simulink model "mloc_diag_vehicle"  (R2018b)
settings: configuration reference "Active" (kept outside this file)
undefined symbols (not defined in the file): P_MLOC_ActivateVehicleUnstableDetection_b, P_MLOC_BetaMax_rad, P_MLOC_SafeStandstill_FMax_N, P_MLOC_SafeStandstill_vabsMax_mps
libraries: simulink x3
settings Model: DataDictionary=mloc_diag_vehicle.sldd  Creator=wischnewski  LastModifiedBy=ge34qer

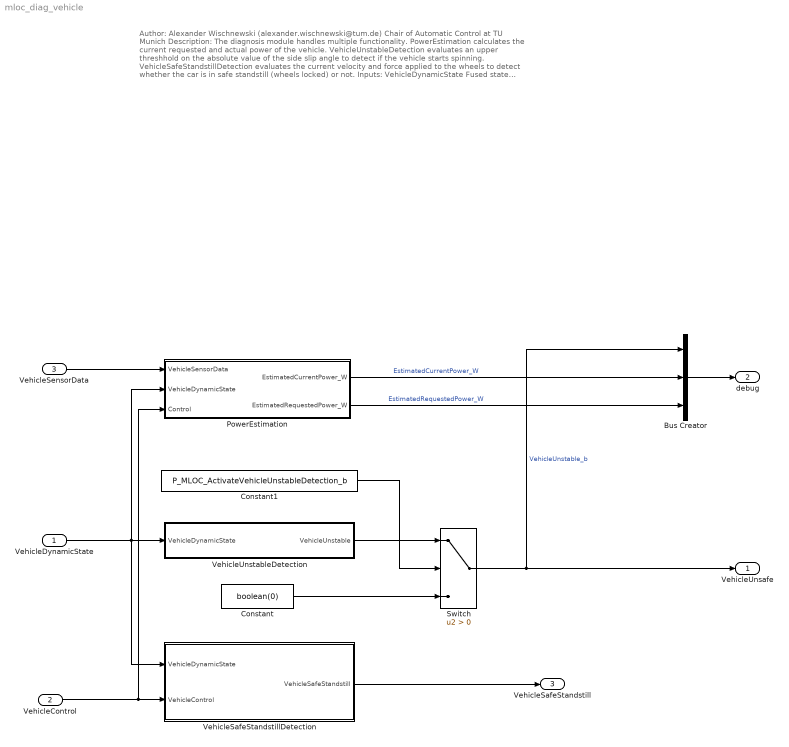
== system mloc_diag_vehicle ==
  note: Author: Alexander Wischnewski (alexander.wischnewski@tum.de)
      | Chair of Automatic Control at TU Munich
      |
      | Description: The diagnosis module handles multiple functionality.
      |
      | PowerEstimation calculates the current requested and actual power of the
      | vehicle.
      |
      | VehicleUnstableDetection evaluates an upper threshhold on the absolute value
      | of the side slip angle to detect if the vehicle starts spinning.
      |
      | VehicleSafeStandstillDetection evaluates the current velocity and force applied to the
      | wheels to detect whether the car is in safe standstill (wheels locked) or not.
      |
      | Inputs:
      | VehicleDynamicState Fused state vector of the vehicle (including position, velocity, acceleration, etc.)
      | VehicleControl Low level vehicle controller output
      | VehicleSensorData Raw sensor data of all vehicle sensors
      |
      | Outputs:
      | debug All debug values
      | VehicleUnsafe Safety critical diagnosis triggered
      | VehicleSafeStandstill Safe standstill detected
  "VehicleDynamicState " : Inport  OutDataTypeStr=Bus: VehicleDynamicState
  VehicleControl : Inport  Port=2  OutDataTypeStr=Bus: VehicleControl
  VehicleSensorData : Inport  Port=3  OutDataTypeStr=Bus: VehicleSensorData
  Bus Creator : BusCreator  Inputs=3  OutDataTypeStr=Bus: mloc_diag_vehicle_debug
  Constant : Constant  Value=boolean(0)
  Constant1 : Constant  Value=P_MLOC_ActivateVehicleUnstableDetection_b
  PowerEstimation : Subsystem
  Switch : Switch  Criteria=u2 > Threshold
  VehicleSafeStandstillDetection : Subsystem
  VehicleUnstableDetection : Subsystem
  VehicleUnsafe : Outport  OutDataTypeStr=boolean
  debug : Outport  Port=2  OutDataTypeStr=Bus: mloc_diag_vehicle_debug
  VehicleSafeStandstill : Outport  Port=3  OutDataTypeStr=boolean
  wires:
  "VehicleDynamicState "/1 -> PowerEstimation/2(VehicleDynamicState), VehicleSafeStandstillDetection/1(VehicleDynamicState), VehicleUnstableDetection/1(VehicleDynamicState)
  VehicleUnstableDetection/1(VehicleUnstable) -> Switch/1
  Switch/1 -> VehicleUnsafe/1, Bus Creator/1  "VehicleUnstable_b"
  Constant/1 -> Switch/3
  Constant1/1 -> Switch/2
  Bus Creator/1 -> debug/1
  VehicleSafeStandstillDetection/1(VehicleSafeStandstill) -> VehicleSafeStandstill/1
  VehicleControl/1 -> PowerEstimation/3(Control), VehicleSafeStandstillDetection/2(VehicleControl)
  VehicleSensorData/1 -> PowerEstimation/1(VehicleSensorData)
  PowerEstimation/1(EstimatedCurrentPower_W) -> Bus Creator/2  "EstimatedCurrentPower_W"
  PowerEstimation/2(EstimatedRequestedPower_W) -> Bus Creator/3  "EstimatedRequestedPower_W"

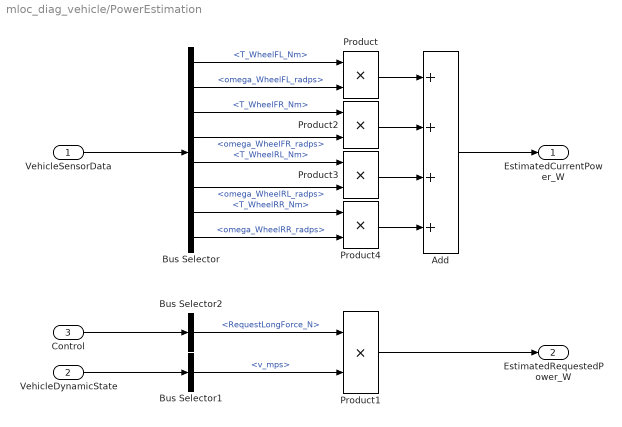
== system mloc_diag_vehicle/PowerEstimation ==
  VehicleSensorData : Inport
  VehicleDynamicState : Inport  Port=2
  Control : Inport  Port=3
  Add : Sum  Inputs=4
  Bus Selector : BusSelector  OutputSignals=T_WheelFL_Nm,omega_WheelFL_radps,T_WheelFR_Nm,omega_WheelFR_radps,T_WheelRL_Nm,omega_WheelRL_radps,T_WheelRR_Nm,omega_WheelRR_radps
  Bus Selector1 : BusSelector  OutputSignals=v_mps
  Bus Selector2 : BusSelector  OutputSignals=RequestLongForce_N
  Product{,1..4} (5 alike) : Product
  EstimatedCurrentPower_W : Outport
  EstimatedRequestedPower_W : Outport  Port=2
  wires:
  Product1/1 -> EstimatedRequestedPower_W/1
  Control/1 -> Bus Selector2/1
  Bus Selector2/1 -> Product1/1  "<RequestLongForce_N>"
  VehicleDynamicState/1 -> Bus Selector1/1
  Bus Selector1/1 -> Product1/2  "<v_mps>"
  VehicleSensorData/1 -> Bus Selector/1
  Bus Selector/1 -> Product/1  "<T_WheelFL_Nm>"
  Bus Selector/2 -> Product/2  "<omega_WheelFL_radps>"
  Bus Selector/3 -> Product2/1  "<T_WheelFR_Nm>"
  Bus Selector/4 -> Product2/2  "<omega_WheelFR_radps>"
  Bus Selector/5 -> Product3/1  "<T_WheelRL_Nm>"
  Bus Selector/6 -> Product3/2  "<omega_WheelRL_radps>"
  Bus Selector/7 -> Product4/1  "<T_WheelRR_Nm>"
  Bus Selector/8 -> Product4/2  "<omega_WheelRR_radps>"
  Product/1 -> Add/1
  Product2/1 -> Add/2
  Product3/1 -> Add/3
  Product4/1 -> Add/4
  Add/1 -> EstimatedCurrentPower_W/1

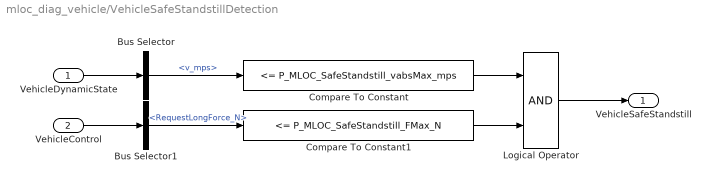
== system mloc_diag_vehicle/VehicleSafeStandstillDetection ==
  VehicleDynamicState : Inport
  VehicleControl : Inport  Port=2
  Bus Selector : BusSelector  OutputSignals=v_mps
  Bus Selector1 : BusSelector  OutputSignals=RequestLongForce_N
  Compare To Constant : simulink/Logic and Bit Operations/Compare To Constant  relop=<=  const=P_MLOC_SafeStandstill_vabsMax_mps  OutDataTypeStr=boolean
  Compare To Constant1 : simulink/Logic and Bit Operations/Compare To Constant  relop=<=  const=P_MLOC_SafeStandstill_FMax_N  OutDataTypeStr=boolean
  Logical Operator : Logic  AllPortsSameDT=off  OutDataTypeStr=boolean
  VehicleSafeStandstill : Outport
  wires:
  VehicleDynamicState/1 -> Bus Selector/1
  Bus Selector/1 -> Compare To Constant/1  "<v_mps>"
  Compare To Constant/1 -> Logical Operator/1
  Compare To Constant1/1 -> Logical Operator/2
  Logical Operator/1 -> VehicleSafeStandstill/1
  VehicleControl/1 -> Bus Selector1/1
  Bus Selector1/1 -> Compare To Constant1/1  "<RequestLongForce_N>"

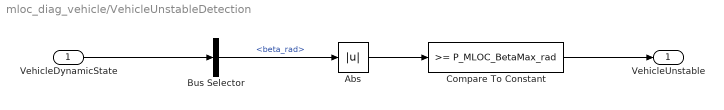
== system mloc_diag_vehicle/VehicleUnstableDetection ==
  VehicleDynamicState : Inport
  Abs : Abs
  Bus Selector : BusSelector  OutputSignals=beta_rad
  Compare To Constant : simulink/Logic and Bit Operations/Compare To Constant  relop=>=  const=P_MLOC_BetaMax_rad  OutDataTypeStr=boolean
  VehicleUnstable : Outport
  wires:
  VehicleDynamicState/1 -> Bus Selector/1
  Bus Selector/1 -> Abs/1  "<beta_rad>"
  Compare To Constant/1 -> VehicleUnstable/1
  Abs/1 -> Compare To Constant/1
